simulink model "sampleModel1889_5"  (R2023a)
settings: Solver=VariableStepAuto  StartTime=0.0  StopTime=10.0  RelTol=1e-3
libraries: hdlsllib x8, simulink x4
settings Model: Creator=user1  LastModifiedBy=user1

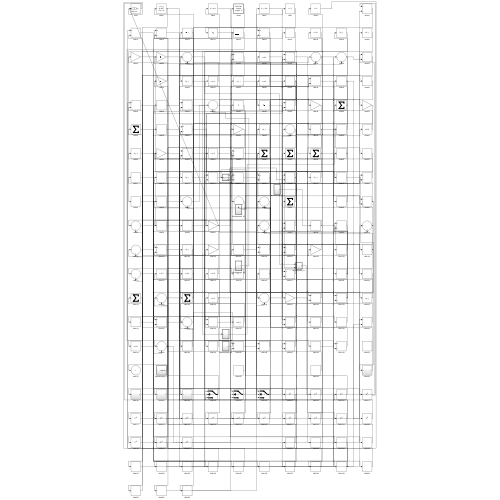
[thumbnail: Simulink's stored preview of the top-level diagram]
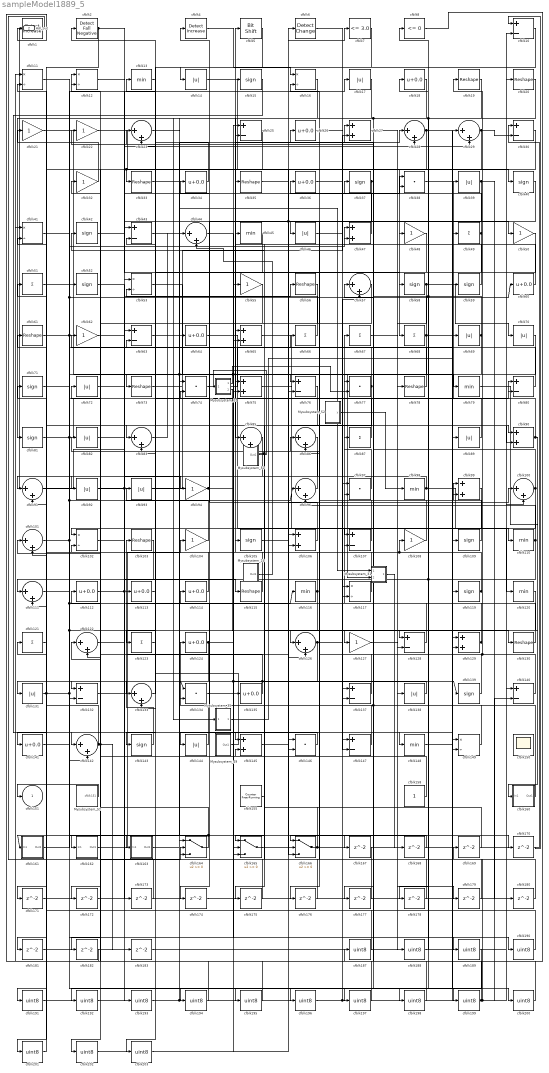
== system sampleModel1889_5 ==
  Mysubsystem_12 : Subsystem  TreatAsAtomicUnit=on  RTWFcnName=Mysubsystem_12
      settings: RTWFcnNameOpts=User specified  RTWFileNameOpts=Use function name
  Mysubsystem_24 : Subsystem  TreatAsAtomicUnit=on  RTWFcnName=Mysubsystem_24
      settings: RTWFcnNameOpts=User specified  RTWFileNameOpts=Use function name
  Mysubsystem_31 : Subsystem  TreatAsAtomicUnit=on  RTWFcnName=Mysubsystem_31
      settings: RTWFcnNameOpts=User specified  RTWFileNameOpts=Use function name
  Mysubsystem_35 : Subsystem  TreatAsAtomicUnit=on  RTWFcnName=Mysubsystem_35
      settings: RTWFcnNameOpts=User specified  RTWFileNameOpts=Use function name
  Mysubsystem_49 : Subsystem  TreatAsAtomicUnit=on  RTWFcnName=Mysubsystem_49
      settings: RTWFcnNameOpts=User specified  RTWFileNameOpts=Use function name
  Mysubsystem_50 : Subsystem  TreatAsAtomicUnit=on  RTWFcnName=Mysubsystem_50
      settings: RTWFcnNameOpts=User specified  RTWFileNameOpts=Use function name
  Mysubsystem_51 : Subsystem  TreatAsAtomicUnit=on  RTWFcnName=Mysubsystem_51
      settings: RTWFcnNameOpts=User specified  RTWFileNameOpts=Use function name
  Mysubsystem_52 : Subsystem  TreatAsAtomicUnit=on  RTWFcnName=Mysubsystem_52
      settings: RTWFcnNameOpts=User specified  RTWFileNameOpts=Use function name
  cfblk1 : simulink/Logic and Bit Operations/Detect Increase  vinit=0.0  OutDataTypeStr=uint8
      settings: LibrarySourceBlock=|
      | hdlsllib/Logic and Bit
      | Operations/Detect
      | Increase
  cfblk{10,25,30,43,63,76,80,107,128,132,137,140,147} (13 alike) : Sum  Inputs=+-  OutDataTypeStr=uint8
  cfblk{23,28..29,44,57,83,85..86,91,96,100..101,111,122,126,133,142} (17 alike) : Sum  Inputs=|++  OutDataTypeStr=uint8
  cfblk{11..12,16,41,53,102,117,149} (8 alike) : Product  Inputs=*/  OutDataTypeStr=uint8  RndMeth=Zero  SaturateOnIntegerOverflow=on
  cfblk{19..20,33,35,56,61,73,78,103,115,130} (11 alike) : Reshape
  cfblk{21..22,32,48,50,55,62,94,104,108,127} (11 alike) : Gain  OutDataTypeStr=uint8
  cfblk{15,37,40,42,52,58..59,71,81,105,109,119,139,143} (14 alike) : Signum
  cfblk{27,47,65,75,90,99,106,129,145} (9 alike) : Sum  OutDataTypeStr=uint8
  cfblk{13,45,79,98,110,116,120,148} (8 alike) : MinMax  OutDataTypeStr=uint8
  cfblk{18,26,34,36,60,64,112..114,124,135,141} (12 alike) : Bias  Bias=0.0  SaturateOnIntegerOverflow=off
  cfblk{49,51,66..68,87,121,123} (8 alike) : Sum  Inputs=+  OutDataTypeStr=uint8
  cfblk{14,17,39,46,69..70,72,82,89,92..93,131,138,144} (14 alike) : Abs  OutDataTypeStr=uint8  SaturateOnIntegerOverflow=off
  cfblk{38,74,77,97,134,146} (6 alike) : DotProduct  OutDataTypeStr=uint8
  cfblk150 : Scope
      settings: Floating=on
  cfblk155 : hdlsllib/Sources/Counter Free-Running  NumBits=16  tsamp=-1
  cfblk158 : Constant  OutDataTypeStr=uint8  SampleTime=-1
  cfblk160 : Subsystem
      settings: LibrarySourceBlock=|
      | hdlsllib/Ports &
      | Subsystems/Subsystem
  cfblk161 : Subsystem
      settings: LibrarySourceBlock=|
      | hdlsllib/Ports &
      | Subsystems/Subsystem
  cfblk162 : Subsystem
      settings: LibrarySourceBlock=|
      | hdlsllib/Ports &
      | Subsystems/Subsystem
  cfblk163 : Subsystem
      settings: LibrarySourceBlock=|
      | hdlsllib/Ports &
      | Subsystems/Subsystem
  cfblk164 : Switch  OutDataTypeStr=uint8  SaturateOnIntegerOverflow=off  InputSameDT=off
  cfblk165 : Switch  OutDataTypeStr=uint8  SaturateOnIntegerOverflow=off  InputSameDT=off
  cfblk166 : Switch  OutDataTypeStr=uint8  SaturateOnIntegerOverflow=off  InputSameDT=off
  cfblk{167..183} (17 alike) : Delay  SampleTime=1
  cfblk{187..203} (17 alike) : DataTypeConversion  OutDataTypeStr=uint8  SaturateOnIntegerOverflow=off  RndMeth=Floor
  cfblk2 : hdlsllib/Logic and Bit Operations/Detect Fall Negative  vinit=0  OutDataTypeStr=uint8
  cfblk4 : simulink/Logic and Bit Operations/Detect Increase  vinit=0.0  OutDataTypeStr=uint8
      settings: LibrarySourceBlock=|
      | hdlsllib/Logic and Bit
      | Operations/Detect
      | Increase
  cfblk5 : hdlsllib/Logic and Bit Operations/Bit Shift  mode=Shift Left Logical  N=0
  cfblk6 : simulink/Logic and Bit Operations/Detect Change  vinit=0  OutDataTypeStr=uint8
      settings: LibrarySourceBlock=|
      | hdlsllib/Logic and Bit
      | Operations/Detect
      | Change
  cfblk7 : hdlsllib/Logic and Bit Operations/Compare To Constant  relop=<=  const=3.0  OutDataTypeStr=uint8
  cfblk8 : hdlsllib/Logic and Bit Operations/Compare To Zero  relop=<=  OutDataTypeStr=uint8
  cfblk151 : Outport  OutDataTypeStr=uint8  VectorParamsAs1DForOutWhenUnconnected=off
  Hdl_out : Outport  Port=2  OutDataTypeStr=uint8
  wires:
  cfblk162/1(Out1) -> cfblk104/1
  cfblk64/1 -> cfblk110/1
  cfblk17/1 -> cfblk81/1
  cfblk79/1 -> cfblk126/1
  cfblk83/1 -> cfblk44/1
  cfblk15/1 -> cfblk142/1
  cfblk126/1 -> cfblk57/2, cfblk171/1
  cfblk98/1 -> cfblk91/1, cfblk120/1
  cfblk146/1 -> cfblk144/1
  cfblk106/1 -> cfblk34/1
  cfblk164/1 -> cfblk72/1, cfblk161/1(In1)
  cfblk142/1 -> cfblk182/1, cfblk183/1, cfblk121/1
  cfblk1/1 -> cfblk164/2
  cfblk7/1 -> cfblk143/1
  cfblk114/1 -> cfblk71/1
  cfblk78/1 -> cfblk4/1
  cfblk10/1 -> cfblk83/1
  cfblk97/1 -> cfblk67/1
  cfblk143/1 -> cfblk103/1
  cfblk158/1 -> cfblk101/1
  cfblk117/1 -> cfblk5/1
  cfblk144/1 -> cfblk124/1
  cfblk141/1 -> cfblk47/1
  cfblk13/1 -> cfblk123/1
  cfblk81/1 -> cfblk129/2, cfblk195/1, cfblk10/2
  cfblk124/1 -> cfblk131/1, cfblk190/1
  cfblk90/1 -> cfblk39/1, cfblk160/1(In1)
  cfblk16/1 -> cfblk85/1
  cfblk59/1 -> cfblk35/1
  cfblk160/1(Out1) -> cfblk27/1, cfblk66/1
  cfblk2/1 -> cfblk91/2, cfblk58/1
  cfblk47/1 -> cfblk36/1
  cfblk48/1 -> cfblk73/1
  cfblk89/1 -> cfblk43/2
  cfblk14/1 -> cfblk68/1
  cfblk148/1 -> cfblk29/1
  cfblk130/1 -> cfblk87/1
  cfblk40/1 -> cfblk76/2, cfblk174/1
  cfblk5/1 -> cfblk14/1
  cfblk105/1 -> cfblk7/1
  cfblk103/1 -> cfblk111/1
  cfblk11/1 -> cfblk199/1
  cfblk32/1 -> cfblk21/1
  cfblk129/1 -> cfblk19/1, cfblk97/2
  cfblk140/1 -> cfblk82/1, cfblk99/2
  cfblk25/1 -> cfblk33/1, cfblk201/1
  cfblk58/1 -> cfblk70/1, cfblk128/2
  cfblk29/1 -> cfblk102/1, cfblk30/2
  cfblk28/1 -> cfblk90/1, cfblk181/1
  cfblk34/1 -> cfblk2/1
  cfblk82/1 -> cfblk130/1
  cfblk20/1 -> cfblk191/1
  cfblk123/1 -> cfblk53/2
  cfblk110/1 -> cfblk162/1(In1), cfblk198/1, cfblk96/2
  cfblk132/1 -> cfblk6/1
  cfblk43/1 -> cfblk145/1, cfblk75/2
  cfblk42/1 -> cfblk29/2
  cfblk80/1 -> cfblk47/2
  cfblk71/1 -> cfblk65/1
  cfblk163/1(Out1) -> cfblk28/1
  cfblk21/1 -> cfblk138/1
  cfblk44/1 -> cfblk135/1
  cfblk46/1 -> cfblk117/1
  cfblk75/1 -> cfblk119/1
  cfblk72/1 -> cfblk127/1
  cfblk69/1 -> Mysubsystem_31/2(In2), cfblk18/1, cfblk25/2
  cfblk91/1 -> cfblk17/1
  cfblk22/1 -> cfblk78/1
  cfblk100/1 -> cfblk147/2, cfblk57/1
  cfblk4/1 -> cfblk16/1
  cfblk134/1 -> cfblk80/1, cfblk139/1
  cfblk128/1 -> cfblk113/1
  cfblk93/1 -> cfblk25/1
  cfblk116/1 -> cfblk105/1, cfblk165/1
  cfblk73/1 -> cfblk27/2
  cfblk135/1 -> cfblk32/1, cfblk134/1
  cfblk86/1 -> cfblk92/1
  cfblk102/1 -> cfblk115/1
  cfblk101/1 -> cfblk52/1, cfblk149/2
  cfblk166/1 -> cfblk30/1, cfblk75/1
  cfblk65/1 -> cfblk90/2
  cfblk6/1 -> cfblk79/1
  cfblk38/1 -> cfblk129/1
  cfblk161/1(Out1) -> cfblk60/1, cfblk15/1
  cfblk19/1 -> cfblk134/2, cfblk107/1, cfblk178/1
  cfblk56/1 -> cfblk146/2
  cfblk139/1 -> cfblk37/1
  cfblk68/1 -> cfblk132/2, cfblk165/3, cfblk22/1, cfblk200/1
  cfblk52/1 -> cfblk94/1
  cfblk113/1 -> cfblk163/1(In1)
  cfblk61/1 -> cfblk63/2, cfblk166/3
  cfblk138/1 -> cfblk133/1
  cfblk155/1 -> cfblk85/2, cfblk45/1
  cfblk26/1 -> cfblk137/1
  cfblk37/1 -> cfblk176/1, cfblk197/1
  cfblk30/1 -> cfblk106/2
  cfblk27/1 -> cfblk40/1
  cfblk77/1 -> cfblk111/2, cfblk12/2
  cfblk165/1 -> cfblk28/2
  cfblk70/1 -> cfblk117/2
  cfblk109/1 -> cfblk74/2
  cfblk107/1 -> cfblk62/1
  cfblk119/1 -> cfblk108/1, cfblk12/1, cfblk99/1
  cfblk45/1 -> cfblk65/2
  cfblk74/1 -> cfblk59/1
  cfblk111/1 -> cfblk142/2
  cfblk87/1 -> cfblk26/1
  cfblk121/1 -> cfblk141/1
  cfblk120/1 -> cfblk137/2
  cfblk36/1 -> cfblk48/1
  cfblk63/1 -> cfblk89/1
  cfblk104/1 -> cfblk83/2
  cfblk145/1 -> cfblk100/1
  cfblk137/1 -> cfblk23/1
  cfblk108/1 -> cfblk77/1
  cfblk35/1 -> cfblk50/1
  cfblk131/1 -> cfblk80/2, cfblk96/1, cfblk116/1, cfblk194/1, cfblk61/1
  cfblk85/1 -> cfblk101/2
  cfblk147/1 -> cfblk86/1
  cfblk149/1 -> cfblk114/1
  cfblk133/1 -> cfblk93/1
  cfblk99/1 -> cfblk132/1
  cfblk60/1 -> cfblk49/1
  cfblk94/1 -> cfblk38/1, Hdl_out/1
  cfblk115/1 -> cfblk13/1
  cfblk92/1 -> cfblk148/1, cfblk38/2
  cfblk66/1 -> cfblk23/2
  cfblk12/1 -> cfblk46/1
  cfblk96/1 -> cfblk42/1
  cfblk49/1 -> cfblk133/2, cfblk16/2
  cfblk53/1 -> cfblk166/2
  cfblk112/1 -> cfblk56/1, cfblk167/1
  cfblk39/1 -> cfblk76/1, cfblk180/1
  cfblk167/1 -> cfblk164/3
  cfblk168/1 -> cfblk166/1
  cfblk169/1 -> cfblk146/1
  cfblk23/1 -> cfblk170/1
  cfblk170/1 -> cfblk10/1
  cfblk171/1 -> cfblk43/1
  cfblk57/1 -> cfblk172/1
  cfblk172/1 -> cfblk140/1
  cfblk62/1 -> cfblk173/1
  cfblk173/1 -> cfblk63/1
  cfblk174/1 -> cfblk106/1
  cfblk76/1 -> cfblk175/1
  cfblk175/1 -> cfblk164/1
  cfblk176/1 -> cfblk102/2
  cfblk50/1 -> cfblk177/1
  cfblk177/1 -> cfblk53/1
  cfblk178/1 -> cfblk145/2
  cfblk67/1 -> cfblk179/1
  cfblk179/1 -> cfblk147/1
  cfblk180/1 -> cfblk86/2
  cfblk181/1 -> cfblk165/2
  cfblk182/1 -> cfblk1/1
  cfblk183/1 -> cfblk100/2
  cfblk8/1 -> cfblk187/1
  cfblk187/1 -> cfblk112/1
  cfblk127/1 -> cfblk188/1
  cfblk188/1 -> cfblk8/1
  cfblk51/1 -> cfblk189/1
  cfblk190/1 -> cfblk51/1
  cfblk191/1 -> cfblk149/1, cfblk97/1, cfblk64/1
  cfblk189/1 -> cfblk192/1
  cfblk192/1 -> cfblk20/1
  cfblk122/1 -> cfblk193/1
  cfblk193/1 -> cfblk74/1
  cfblk194/1 -> cfblk122/1
  cfblk195/1 -> cfblk122/2
  cfblk41/1 -> cfblk196/1
  cfblk196/1 -> cfblk109/1
  cfblk197/1 -> cfblk41/1
  cfblk198/1 -> cfblk41/2
  cfblk199/1 -> cfblk169/1, cfblk140/2, cfblk107/2
  cfblk200/1 -> cfblk11/1
  cfblk201/1 -> cfblk11/2
  cfblk55/1 -> cfblk202/1
  cfblk202/1 -> cfblk126/2
  cfblk203/1 -> cfblk55/1
  Mysubsystem_12/1(Out1) -> cfblk77/2
  Mysubsystem_12/2(Out2) -> cfblk128/1
  Mysubsystem_24/1(Out1) -> cfblk44/2
  cfblk33/1 -> Mysubsystem_31/1(In1)
  Mysubsystem_31/1(Out1) -> cfblk168/1
  cfblk18/1 -> Mysubsystem_35/1(In1)
  Mysubsystem_35/1(Out1) -> cfblk69/1
  Mysubsystem_49/1(Out1) -> cfblk203/1
  Mysubsystem_50/1(Out1) -> Mysubsystem_12/1(In1)
  Mysubsystem_51/1(cfblk151) -> cfblk151/1
  Mysubsystem_52/1(y) -> cfblk98/1

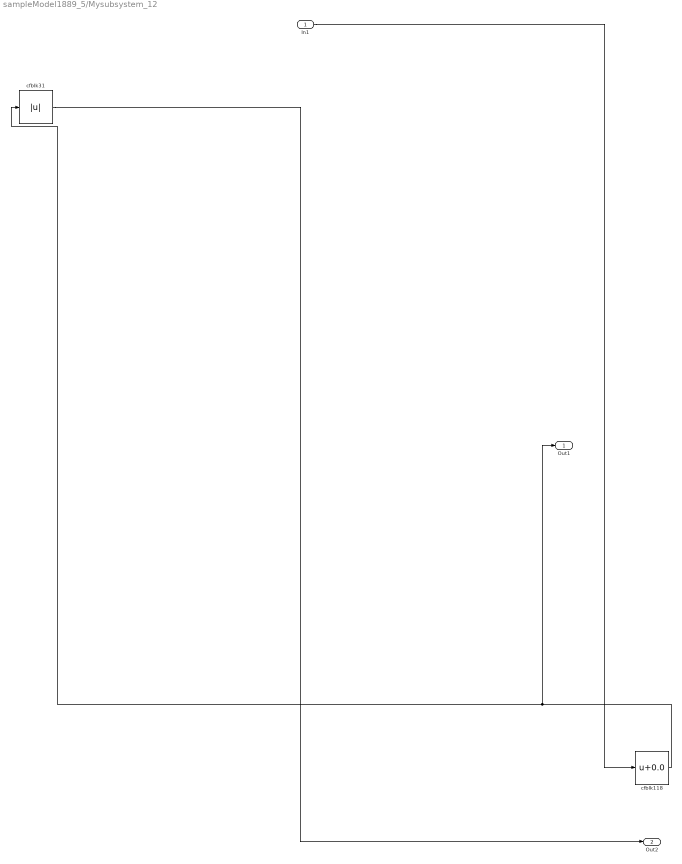
== system sampleModel1889_5/Mysubsystem_12 ==
  In1 : Inport
  cfblk118 : Bias  Bias=0.0  SaturateOnIntegerOverflow=off
  cfblk31 : Abs  SaturateOnIntegerOverflow=off
  Out1 : Outport
  Out2 : Outport  Port=2
  wires:
  cfblk118/1 -> Out1/1, cfblk31/1
  cfblk31/1 -> Out2/1
  In1/1 -> cfblk118/1

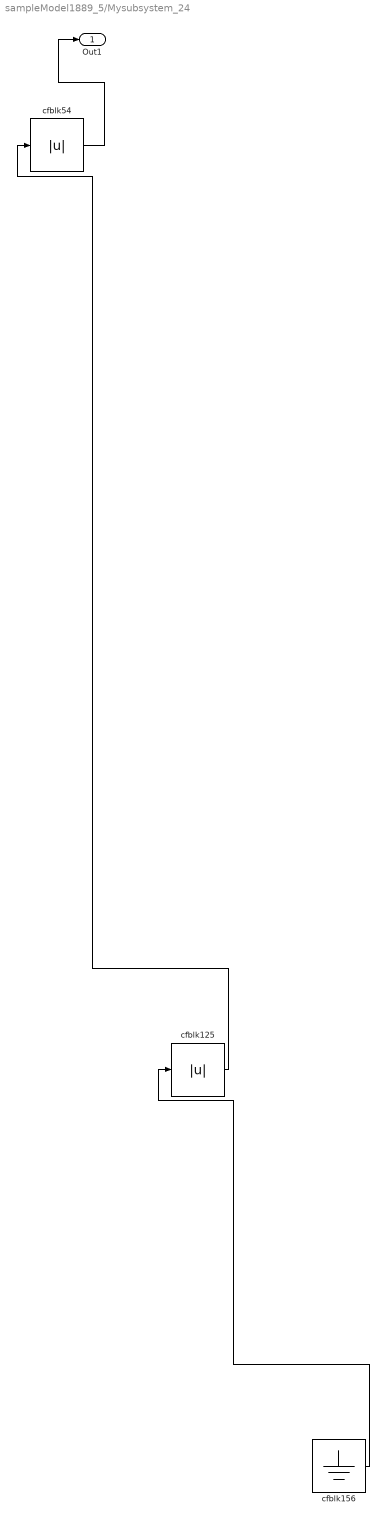
== system sampleModel1889_5/Mysubsystem_24 ==
  cfblk125 : Abs  SaturateOnIntegerOverflow=off
  cfblk156 : Ground
  cfblk54 : Abs  SaturateOnIntegerOverflow=off
  Out1 : Outport
  wires:
  cfblk156/1 -> cfblk125/1
  cfblk125/1 -> cfblk54/1
  cfblk54/1 -> Out1/1

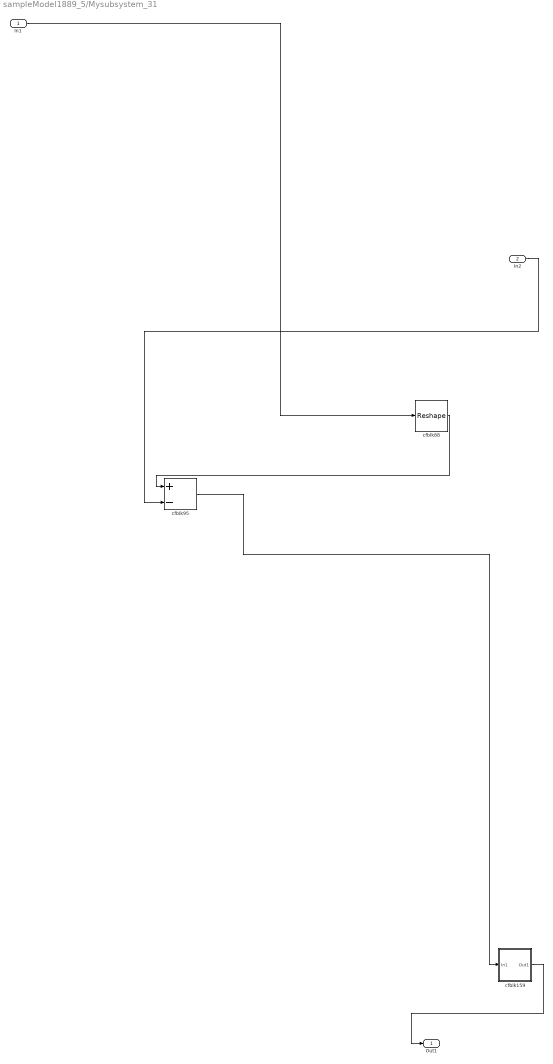
== system sampleModel1889_5/Mysubsystem_31 ==
  In1 : Inport
  In2 : Inport  Port=2
  cfblk159 : Subsystem
      settings: LibrarySourceBlock=|
      | hdlsllib/Ports &
      | Subsystems/Subsystem
  cfblk88 : Reshape
  cfblk95 : Sum  Inputs=+-
  Out1 : Outport
  wires:
  cfblk88/1 -> cfblk95/1
  cfblk95/1 -> cfblk159/1(In1)
  In1/1 -> cfblk88/1
  In2/1 -> cfblk95/2
  cfblk159/1(Out1) -> Out1/1

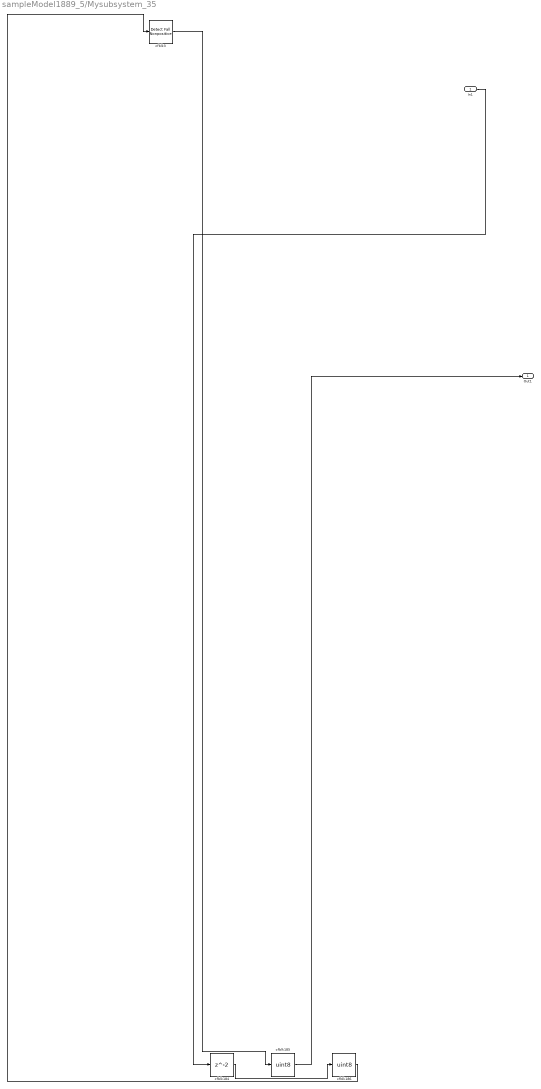
== system sampleModel1889_5/Mysubsystem_35 ==
  In1 : Inport
  cfblk184 : Delay  SampleTime=1
  cfblk185 : DataTypeConversion  OutDataTypeStr=uint8  SaturateOnIntegerOverflow=off  RndMeth=Floor
  cfblk186 : DataTypeConversion  OutDataTypeStr=uint8  SaturateOnIntegerOverflow=off  RndMeth=Floor
  cfblk3 : hdlsllib/Logic and Bit Operations/Detect Fall Nonpositive  vinit=0  OutDataTypeStr=boolean
  Out1 : Outport
  wires:
  cfblk186/1 -> cfblk3/1
  In1/1 -> cfblk184/1
  cfblk184/1 -> cfblk186/1
  cfblk185/1 -> Out1/1
  cfblk3/1 -> cfblk185/1

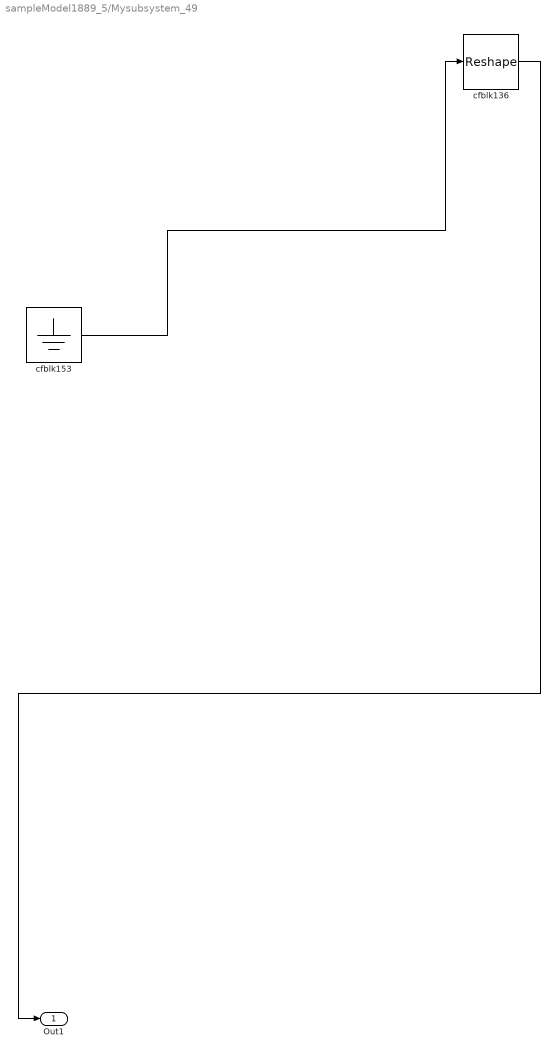
== system sampleModel1889_5/Mysubsystem_49 ==
  cfblk136 : Reshape
  cfblk153 : Ground
  Out1 : Outport
  wires:
  cfblk153/1 -> cfblk136/1
  cfblk136/1 -> Out1/1

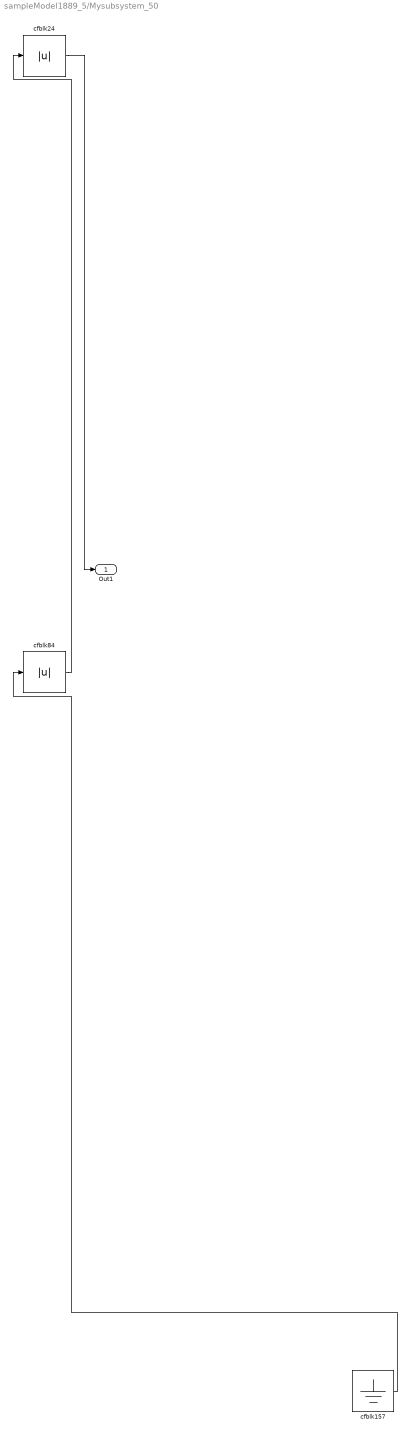
== system sampleModel1889_5/Mysubsystem_50 ==
  cfblk157 : Ground
  cfblk24 : Abs  SaturateOnIntegerOverflow=off
  cfblk84 : Abs  SaturateOnIntegerOverflow=off
  Out1 : Outport
  wires:
  cfblk84/1 -> cfblk24/1
  cfblk157/1 -> cfblk84/1
  cfblk24/1 -> Out1/1

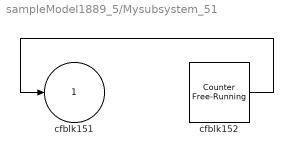
== system sampleModel1889_5/Mysubsystem_51 ==
  cfblk152 : hdlsllib/Sources/Counter Free-Running  NumBits=16  tsamp=-1
  cfblk151 : Outport  VectorParamsAs1DForOutWhenUnconnected=off
  wires:
  cfblk152/1 -> cfblk151/1

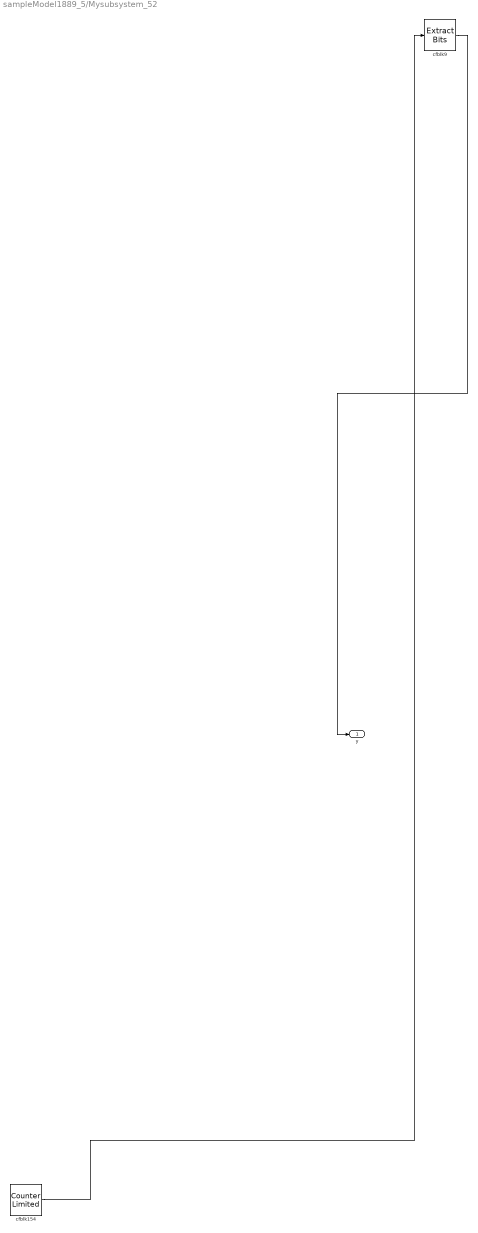
== system sampleModel1889_5/Mysubsystem_52 ==
  cfblk154 : hdlsllib/Sources/Counter Limited  uplimit=7  tsamp=-1
  cfblk9 : simulink/Logic and Bit Operations/Extract Bits  bitsToExtract=Upper half  numBits=8  bitIdxRange=[0 7]  outScalingMode=Preserve fixed-point scaling
      settings: LibrarySourceBlock=|
      | hdlsllib/Logic and Bit
      | Operations/Extract Bits
  y : Outport
  wires:
  cfblk154/1 -> cfblk9/1
  cfblk9/1 -> y/1

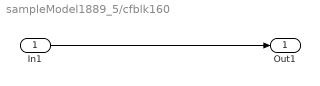
== system sampleModel1889_5/cfblk160 ==
  In1 : Inport
  Out1 : Outport
  wires:
  In1/1 -> Out1/1

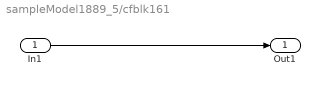
== system sampleModel1889_5/cfblk161 ==
  In1 : Inport
  Out1 : Outport
  wires:
  In1/1 -> Out1/1

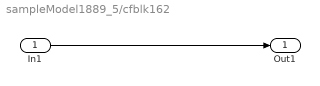
== system sampleModel1889_5/cfblk162 ==
  In1 : Inport
  Out1 : Outport
  wires:
  In1/1 -> Out1/1

== system sampleModel1889_5/cfblk163 ==
  In1 : Inport
  Out1 : Outport
  wires:
  In1/1 -> Out1/1

== system sampleModel1889_5/Mysubsystem_31/cfblk159 ==
  In1 : Inport
  Out1 : Outport
  wires:
  In1/1 -> Out1/1
